simulink model "astron_hw_test_au50_64k"  (R2021a)
settings: Solver=VariableStepDiscrete  StartTime=0.0  StopTime=2048  RelTol=1e-3
undefined symbols (not defined in the file): d0, d1, d2, d3, FFT, sr, Wideband_FFT
libraries: xbsIndex_r4 x637, casper_library_misc x4, xps_library x1
(part 3 of 14)

== system astron_hw_test_au50_64k/bram_in1 ==
  addr : Inport
  data_in : Inport  Port=2
  we : Inport  Port=3
  Terminator : Terminator
  Terminator1 : Terminator
  Terminator2 : Terminator
  astron_hw_test_au50_64k_bram_in1_addr : xbsIndex_r4/Gateway Out  inherit_from_input=off  hdl_port=on  rows=1  columns=1  UseAsDAC=off  DACChannel='1'  interface=None  automatic_assignment=on  address_offset=hex2dec('00')  intf_name=''  intf_description=''  timing_constraint=None  locs_specified=off  LOCs={'A5','B9','A9','C1','A3','G6','E9','A6','A7','A8','B8','B1','B3','D9','B5','B4','B6','C2'}  io_standard={}  block_type=gatewayout
      settings: infoedit="Gateway out block.  Converts Xilinx fixed point inputs into ouputs of type Simulink integer, double, or fixed point.<P><P>Hardware notes:  In hardware these blocks become top level output ports or are discarded, depending on how they are configured."  sginterface={'Nallatech'=>{'xdspkit'=>{'non_memory_mapped_port'=>'uprev_Shared_BRAM_addr'}},'Xilinx'=>{'jtaghwcosim'=>{'non_memory_mapped_port'=>'uprev_Shared_BRAM_addr'},'xdspkit'=>{'non_memory_mapped_port'=>'uprev_Shared_BRAM_addr'}}}  xl_area=[0, 0, 0, 0, 0, 0, 0]
  astron_hw_test_au50_64k_bram_in1_data_in : xbsIndex_r4/Gateway Out  inherit_from_input=off  hdl_port=on  rows=1  columns=1  UseAsDAC=off  DACChannel='1'  interface=None  automatic_assignment=on  address_offset=hex2dec('00')  intf_name=''  intf_description=''  timing_constraint=None  locs_specified=off  LOCs={'B21','B22','A22','B23','B19','C19','A20','A21','A23','B24','A24','A25','E18','D18','C18','B18'}  io_standard={}  block_type=gatewayout
      settings: infoedit="Gateway out block.  Converts Xilinx fixed point inputs into ouputs of type Simulink integer, double, or fixed point.<P><P>Hardware notes:  In hardware these blocks become top level output ports or are discarded, depending on how they are configured."  sginterface={'Nallatech'=>{'xdspkit'=>{'non_memory_mapped_port'=>'uprev_Shared_BRAM_data_in'}},'Xilinx'=>{'jtaghwcosim'=>{'non_memory_mapped_port'=>'uprev_Shared_BRAM_data_in'},'xdspkit'=>{'non_memory_mapped_port'=>'uprev_Shared_BRAM_data_in'}}}  xl_area=[0, 0, 0, 0, 0, 0, 0]
  astron_hw_test_au50_64k_bram_in1_data_out : xbsIndex_r4/Gateway In  gui_display_data_type=Fixed-point  arith_type=Unsigned  n_bits=32  bin_pt=0  preci_type=Single  exp_width=8  frac_width=24  rows=1  columns=1  quantization=Truncate  overflow=Wrap  period=sample_rate  UseAsADC=off  ADCChannel='1'  interface=None  automatic_assignment=on  address_offset=hex2dec('00')  intf_name=''  intf_description=''  default_value=0  timing_constraint=None  locs_specified=off  LOCs={}  io_standard={}  inherit_from_input=off  hdl_port=on  dbl_ovrd=off  block_type=gatewayin
      settings: xl_area=[0, 0, 0, 0, 0, 0, 0]
  astron_hw_test_au50_64k_bram_in1_we : xbsIndex_r4/Gateway Out  inherit_from_input=off  hdl_port=on  rows=1  columns=1  UseAsDAC=off  DACChannel='1'  interface=None  automatic_assignment=on  address_offset=hex2dec('00')  intf_name=''  intf_description=''  timing_constraint=None  locs_specified=off  LOCs={'A14'}  io_standard={}  block_type=gatewayout
      settings: infoedit="Gateway out block.  Converts Xilinx fixed point inputs into ouputs of type Simulink integer, double, or fixed point.<P><P>Hardware notes:  In hardware these blocks become top level output ports or are discarded, depending on how they are configured."  xl_area=[0, 0, 0, 0, 0, 0, 0]
  calc_add : Subsystem  mask{data_width=32, addr_width=14, sample_rate=sample_rate}
      mask prompts: data_width "data width"; addr_width "address width"; sample_rate "sample rate"
  convert_addr : xbsIndex_r4/Convert  gui_display_data_type=Fixed-point  arith_type=Unsigned  n_bits=addr_width  bin_pt=0  float_type=Single  exp_bits=8  fraction_bits=24  quantization=Truncate  overflow=Wrap  en=off  latency=0  pipeline=off  dbl_ovrd=off  block_type=convert
      settings: xl_area=[0, 0, 0, 0, 0, 0, 0]
  convert_din1 : xbsIndex_r4/Convert  gui_display_data_type=Fixed-point  arith_type=Unsigned  n_bits=32  bin_pt=0  float_type=Single  exp_bits=8  fraction_bits=24  quantization=Truncate  overflow=Wrap  en=off  latency=0  pipeline=off  dbl_ovrd=off  block_type=convert
      settings: xl_area=[0, 0, 0, 0, 0, 0, 0]
  convert_we : xbsIndex_r4/Convert  gui_display_data_type=Fixed-point  arith_type=Unsigned  n_bits=1  bin_pt=0  float_type=Single  exp_bits=8  fraction_bits=24  quantization=Truncate  overflow=Wrap  en=off  latency=0  pipeline=off  dbl_ovrd=off  block_type=convert
      settings: xl_area=[0, 0, 0, 0, 0, 0, 0]
  munge_in : Subsystem  AncestorBlock=casper_library_flow_control/munge  mask(munge){divisions=1, div_size=32, order=[0], arith_type_out=Unsigned, bin_pt_out=0}
      mask prompts: divisions "Number of divisions"; div_size "Division size (bits)"; order "Division packing order"; arith_type_out "Output arithmetic type"; bin_pt_out "Output binary point"
      mask help: Splits an input bus into the specified number of divisions and then recombines them in the order specified (most significant division = 0,least = number divisions-1)
      mask init:
      | munge_init(gcb, ...
      |     'divisions', divisions, ...
      |     'div_size', div_size, ...
      |     'order', order, ...
      |     'arith_type_out', arith_type_out, ...
      |     'bin_pt_out', bin_pt_out);
      settings: AttributesFormatString=|
      | split:32
      | join:0
      | Unsigned [32,0]
      mask TypeOptions arith_type_out: Unsigned | Signed  (2's comp) | Floating-point
  munge_out : Subsystem  AncestorBlock=casper_library_flow_control/munge  mask(munge){divisions=1, div_size=32, order=[0], arith_type_out=Signed  (2's comp), bin_pt_out=0}
      mask prompts: divisions "Number of divisions"; div_size "Division size (bits)"; order "Division packing order"; arith_type_out "Output arithmetic type"; bin_pt_out "Output binary point"
      mask help: Splits an input bus into the specified number of divisions and then recombines them in the order specified (most significant division = 0,least = number divisions-1)
      mask init:
      | munge_init(gcb, ...
      |     'divisions', divisions, ...
      |     'div_size', div_size, ...
      |     'order', order, ...
      |     'arith_type_out', arith_type_out, ...
      |     'bin_pt_out', bin_pt_out);
      settings: AttributesFormatString=|
      | split:32
      | join:0
      | Signed  (2's comp) [32,0]
      mask TypeOptions arith_type_out: Unsigned | Signed  (2's comp) | Floating-point
  sim_mem : Subsystem  mask{arith_type=Signed  (2's comp), addr_width=14, data_width=32, data_bin_pt=0, init_vals=[1984   3085   5930   4112  -1496   3544    264   1678 -11500  -1800   2816    776  -3465   3294   4211   1264   6657  -1429    705  -4034    302   1131  11510  -4445  -3511  -4928  -4006    183    615  12343   2073  -5388  -3380    845  -4164  -1061  -3764   2787  -3852   2474  -2893   3321  -1352  -5924  -3318   9147  -1048   2948   1398  -1169    -41  -7781   2741  -4502  -3047  -4890   4740    976  -2802   1720  -1780   2508   -464  -8281   8910   4106   2850   3611  -5526    885  -3618  -3616  -2938   5662   2713 -12635  -1390   3325   -154   -343  -3020   3434  -8336   3105    857   2550   1784   3008   4311   -201    881  -6122  -1465   3077   4417   4239   1117  -1309   6053   -698  -1071  -1645  -4228  -9855  -2884   3889   -837   3243  -1377   -135   1408   2950  -1868  -3051  -2380    655  -4225   5749   -586   2697  -7881  -6099   2206  -6840    444   -804  -9734  -8880   -597   4783  -7634  -1844   6561   5694  -5544   -857   -730  -2457  -6910  -2128   5936   7001  -3620   -273    353   6624   1431  -1099   -714  -1959  -3555  -6239  -3170   1805   1947    854  -1442  11189   1094  -3682    123   -313   2125  -1304  -6534  -1204   1989   3537  10081   1658   -798  -2051    541   1394   3322    425   3350   1804  -2357  -2617   4959   3829   6155  -6720  -1055   5201   4652  -4609   2781  -8211    173   -235   8718  -5823  -5542  -1330  -3142  -3121  -1370   4064   -961   1860    510  -5034  -1795  -3714   -168   5586   -469   -271  -1197   1706   8129   5634  -6588  -9076   5796   4269    598   1067  -3096   -684 -11313   1929   2411   8778  -9921  -3811   1039    556  -2910  -5552  -1849   2807   4123   3804   4656   2813    948   7339  -5002   5371   7833   -814   6143    359   3754  -4198   7336   3079   5582   2550  -1221  -2554  -5287   1018   3237    462   1840  -8743   -248   4298  -3411  -4165  -6395  -7870  -2522   4693   -822   -725  -4702  -3794   2657   1675  -2382   -303   1402   -530   7362  -2828  -1933   8909   5599   -265   5292   4757  -8979  -5900    211  -2683  -2990     49   7315  -2186  -1155  -9215    333   -975   3303  -2675   9631  -1505 -13279  -1568  -7533   1443  -4806  -6865    516  -2485   5311  -7290   -813  -6915  -9049  -9449   -640   2648   -868  -5374  -9784   1271   4103   1444  -1607   5601   1767   2379   1847   7764   -195   -967  -1699    303  -3463   -341  -2448  -9376  -6614  -1648   5710   8819  -7816    -39   5820  12043  -1350  -3198   4878  -2472   3668  -9660  -1589   6711   4066  -3417   -647   -769   -130    820  -1059  -2005   1501   2484   2933  -9339     67   -279    286   4766  -2646    817   6765    126  -1103    772   4745   2056  -4242  -4808   2507   3274  -3883  -7998   2094   6813  -1839  -1749   2093   3845    226   3291   1916  -1914    497   1824  -4396  -3279  -5275  -5271   2871   7212   -789   -109   2358  -2123    564  -2250  -5137   1800  -3902  -4350  -1511   4172    -19   3743  -5473    903  -6474  -3989   6195    709  -6542  -1685     97   3221  -4414  -2913   9057   1792  -1026  -4029  -1206  10766   4491   2275   3214   1807  -8910    -64   9374   4351  -3176    182   -867   5543  -2676  -5001   -986  -2146   4379   3872   1612   1319  -7989  -2628  -1137   4274  -7967   3856     99   1211   6480  -1088    949   3958  -4649   1153  -6252   5056  -3421  -2594  -6975    860    434   5101  -4961  -1864  -1437  -5845   6867   4257   -826  -2147  -3300   1901  -4196 -11590   2009  -2242   -968   3948    772   1163   -380  -2475   2307   -674   -739  -4259  -4145  -4987   -915   4277   3058   4506  -2795   1237   -819   5321  -2081  -3272  -1469   7910    896  -1396  -3690  -1514   4741   2153  -2699   8800  -1671  -7213   3480   6032  -3929  -2137    868  -4624  -2774  -1098   1304   8720  -3706   3800    787   2834    482  -4352   -735   2706  -3180 -10261   -617  -1053  -2513   2194   8394  -1662   -586  -2273  -4140   9675   2696  -2289  -6628  -2089   6262  -3522  -3956   3670   -443   4494   6253   2300 -11463  -9828   -285   -279  -3345 ...(+110690 chars)], sample_rate=1, csp_latency=1}
      mask prompts: arith_type "Output Data Type"; addr_width "Address width"; data_width "Data width"; data_bin_pt "Data Binary Point"; init_vals "Initial values"; sample_rate "Sample rate"; csp_latency "Latency"
      mask init:
      | % set_param([gcb, '/data_to_xilinx'], 'arith_type', arith_type)
      | % set_param([gcb, '/data_to_xilinx'], 'n_bits', get_param(gcb, 'data_width'))
      mask TypeOptions arith_type: Unsigned | Signed  (2's comp)
      mask TypeOptions data_width: 8 | 16 | 32 | 64 | 128
  data_out : Outport  VectorParamsAs1DForOutWhenUnconnected=off
  wires:
  munge_out/1(dout) -> data_out/1
  sim_mem/1(data_out) -> astron_hw_test_au50_64k_bram_in1_data_out/1
  astron_hw_test_au50_64k_bram_in1_data_out/1 -> munge_out/1(din)
  convert_addr/1 -> astron_hw_test_au50_64k_bram_in1_addr/1
  convert_din1/1 -> astron_hw_test_au50_64k_bram_in1_data_in/1
  data_in/1 -> munge_in/1(din)
  calc_add/1(out) -> convert_addr/1
  astron_hw_test_au50_64k_bram_in1_we/1 -> Terminator2/1
  astron_hw_test_au50_64k_bram_in1_data_in/1 -> Terminator1/1
  astron_hw_test_au50_64k_bram_in1_addr/1 -> Terminator/1
  convert_we/1 -> astron_hw_test_au50_64k_bram_in1_we/1
  addr/1 -> sim_mem/1(addr), calc_add/1(in)
  we/1 -> sim_mem/3(we), convert_we/1
  munge_in/1(dout) -> sim_mem/2(data), convert_din1/1
